simulink model "sampleModel1587"  (R2023a)
settings: Solver=VariableStepAuto  StartTime=0.0  StopTime=10.0  RelTol=1e-3
libraries: hdlsllib x2, simulink x2
settings Model: Creator=user1  LastModifiedBy=user1

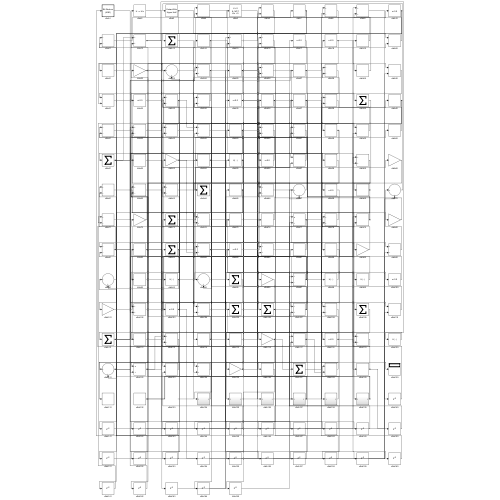
[thumbnail: Simulink's stored preview of the top-level diagram]
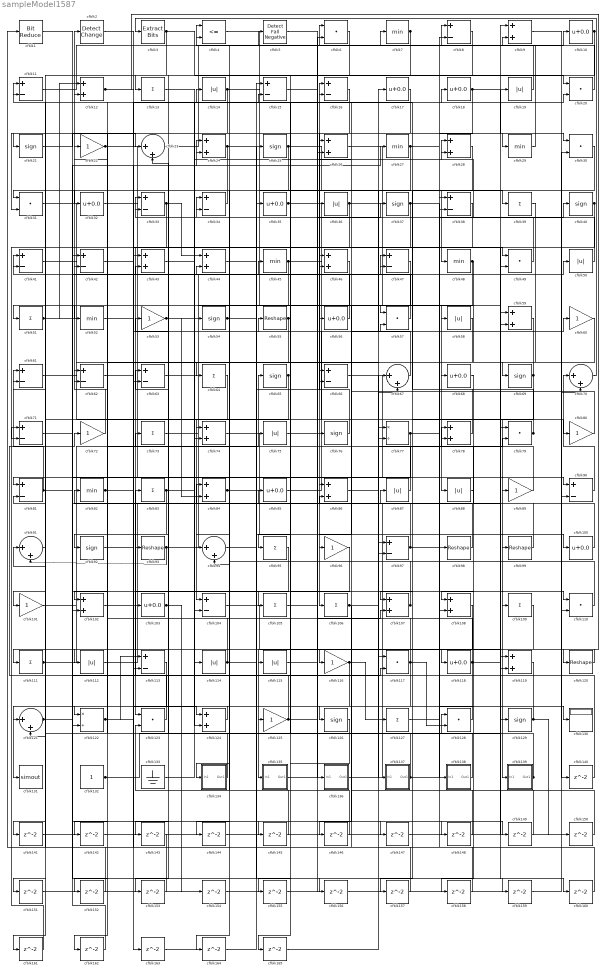
== system sampleModel1587 ==
  cfblk1 : hdlsllib/Logic and Bit Operations/Bit Reduce  mode=AND
  cfblk{10,17..18,32,35,56,68,85,100,103,118} (11 alike) : Bias  Bias=0.0  SaturateOnIntegerOverflow=off
  cfblk{22,53,60,72,80,89,96,101,116,125} (10 alike) : Gain
  cfblk{9,12,24,26,28,43..44,46,59,74,78,84,86,102,107..108,119,124} (18 alike) : Sum
  cfblk{8,11,15..16,33..34,38,41..42,47,61..63,66,71,81,90,97,104,113} (20 alike) : Sum  Inputs=+-
  cfblk{13,39,51,64,73,83,95,105..106,109,111,127} (12 alike) : Sum  Inputs=+
  cfblk{6,20,30..31,49,57,79,110,117,123,128} (11 alike) : DotProduct  OutDataTypeStr=Inherit: Inherit via internal rule
  cfblk{14,19,36,50,58,75,87..88,112,114..115} (11 alike) : Abs  SaturateOnIntegerOverflow=off
  cfblk{55,93,98..99,120} (5 alike) : Reshape
  cfblk{23,67,70,91,94,121} (6 alike) : Sum  Inputs=|++
  cfblk122 : Product  Inputs=*/  RndMeth=Zero  SaturateOnIntegerOverflow=on
  cfblk{21,25,37,40,54,65,69,76,92,126,129} (11 alike) : Signum
  cfblk130 : Display
  cfblk131 : ToWorkspace  VariableName=simout  SaveFormat=Timeseries  SampleTime=-1
  cfblk132 : Constant  SampleTime=-1
  cfblk133 : Ground
  cfblk134 : Subsystem
      settings: LibrarySourceBlock=|
      | hdlsllib/Ports &
      | Subsystems/Subsystem
  cfblk135 : Subsystem
      settings: LibrarySourceBlock=|
      | hdlsllib/Ports &
      | Subsystems/Subsystem
  cfblk136 : Subsystem
      settings: LibrarySourceBlock=|
      | hdlsllib/Ports &
      | Subsystems/Subsystem
  cfblk137 : Subsystem
      settings: LibrarySourceBlock=|
      | hdlsllib/Ports &
      | Subsystems/Subsystem
  cfblk138 : Subsystem
      settings: LibrarySourceBlock=|
      | hdlsllib/Ports &
      | Subsystems/Subsystem
  cfblk139 : Subsystem
      settings: LibrarySourceBlock=|
      | hdlsllib/Ports &
      | Subsystems/Subsystem
  cfblk{140..165} (26 alike) : Delay  SampleTime=1
  cfblk2 : simulink/Logic and Bit Operations/Detect Change  vinit=0  OutDataTypeStr=boolean
      settings: LibrarySourceBlock=|
      | hdlsllib/Logic and Bit
      | Operations/Detect
      | Change
  cfblk{7,27,29,45,48,52,82} (7 alike) : MinMax
  cfblk3 : simulink/Logic and Bit Operations/Extract Bits  bitsToExtract=Upper half  numBits=8  bitIdxRange=[0 7]  outScalingMode=Preserve fixed-point scaling
      settings: LibrarySourceBlock=|
      | hdlsllib/Logic and Bit
      | Operations/Extract Bits
  cfblk4 : RelationalOperator  Operator=<=  OutDataTypeStr=boolean  InputSameDT=off
  cfblk5 : hdlsllib/Logic and Bit Operations/Detect Fall Negative  vinit=0  OutDataTypeStr=boolean
  cfblk77 : Product  Inputs=*/  RndMeth=Zero  SaturateOnIntegerOverflow=on
  wires:
  cfblk33/1 -> cfblk44/1, cfblk52/1
  cfblk14/1 -> cfblk57/1, cfblk31/2
  cfblk87/1 -> cfblk34/1
  cfblk30/1 -> cfblk111/1
  cfblk77/1 -> cfblk81/1, cfblk80/1
  cfblk16/1 -> cfblk106/1
  cfblk139/1(Out1) -> cfblk128/1, cfblk85/1
  cfblk4/1 -> cfblk39/1
  cfblk32/1 -> cfblk90/1
  cfblk26/1 -> cfblk88/1
  cfblk119/1 -> cfblk72/1
  cfblk25/1 -> cfblk134/1(In1), cfblk137/1(In1), cfblk20/2
  cfblk38/1 -> cfblk123/1
  cfblk85/1 -> cfblk60/1
  cfblk76/1 -> cfblk16/1
  cfblk128/1 -> cfblk126/1
  cfblk36/1 -> cfblk58/1, cfblk71/2
  cfblk28/1 -> cfblk48/1
  cfblk111/1 -> cfblk87/1, cfblk27/1, cfblk84/1
  cfblk115/1 -> cfblk76/1
  cfblk27/1 -> cfblk31/1, cfblk29/1
  cfblk43/1 -> cfblk18/1
  cfblk35/1 -> cfblk139/1(In1), cfblk97/2
  cfblk73/1 -> cfblk38/2
  cfblk57/1 -> cfblk11/1
  cfblk129/1 -> cfblk83/1, cfblk150/1
  cfblk125/1 -> cfblk81/2, cfblk107/2
  cfblk70/1 -> cfblk3/1
  cfblk72/1 -> cfblk2/1
  cfblk37/1 -> cfblk130/1, cfblk93/1, cfblk107/1
  cfblk101/1 -> cfblk65/1
  cfblk105/1 -> cfblk47/1
  cfblk65/1 -> cfblk104/1, cfblk94/2
  cfblk117/1 -> cfblk12/2, cfblk128/2, cfblk144/1
  cfblk10/1 -> cfblk95/1, cfblk113/2
  cfblk98/1 -> cfblk45/1
  cfblk104/1 -> cfblk116/1
  cfblk56/1 -> cfblk36/1
  cfblk116/1 -> cfblk127/1, cfblk153/1
  cfblk100/1 -> cfblk78/1
  cfblk8/1 -> cfblk13/1
  cfblk66/1 -> cfblk138/1(In1)
  cfblk13/1 -> cfblk114/1
  cfblk12/1 -> cfblk120/1, cfblk105/1
  cfblk81/1 -> cfblk61/1, cfblk89/1, cfblk145/1
  cfblk91/1 -> cfblk41/1
  cfblk46/1 -> cfblk51/1
  cfblk31/1 -> cfblk104/2
  cfblk53/1 -> cfblk56/1, cfblk84/2
  cfblk113/1 -> cfblk131/1
  cfblk136/1(Out1) -> cfblk9/1
  cfblk132/1 -> cfblk59/1, cfblk6/2
  cfblk89/1 -> cfblk22/1
  cfblk124/1 -> cfblk121/1
  cfblk22/1 -> cfblk119/1, cfblk14/1
  cfblk110/1 -> cfblk15/2
  cfblk7/1 -> cfblk121/2, cfblk143/1
  cfblk108/1 -> cfblk135/1(In1)
  cfblk5/1 -> cfblk136/1(In1)
  cfblk103/1 -> cfblk63/1, cfblk154/1
  cfblk59/1 -> cfblk122/1
  cfblk107/1 -> cfblk82/1, cfblk75/1
  cfblk133/1 -> cfblk28/1
  cfblk67/1 -> cfblk26/1
  cfblk102/1 -> cfblk19/1
  cfblk45/1 -> cfblk59/2, cfblk102/2, cfblk152/1
  cfblk112/1 -> cfblk77/2
  cfblk82/1 -> cfblk124/1, cfblk24/1
  cfblk93/1 -> cfblk57/2, cfblk91/2
  cfblk78/1 -> cfblk47/2
  cfblk60/1 -> cfblk124/2
  cfblk127/1 -> cfblk10/1
  cfblk41/1 -> cfblk43/2
  cfblk2/1 -> cfblk74/1
  cfblk55/1 -> cfblk115/1, cfblk64/1
  cfblk15/1 -> cfblk8/1
  cfblk83/1 -> cfblk54/1, cfblk92/1
  cfblk44/1 -> cfblk86/1
  cfblk135/1(Out1) -> cfblk37/1
  cfblk23/1 -> cfblk7/1
  cfblk50/1 -> cfblk28/2
  cfblk134/1(Out1) -> cfblk62/1
  cfblk58/1 -> cfblk102/1
  cfblk138/1(Out1) -> cfblk53/1
  cfblk63/1 -> cfblk17/1
  cfblk75/1 -> cfblk118/1
  cfblk18/1 -> cfblk63/2, cfblk30/1
  cfblk90/1 -> cfblk70/1
  cfblk3/1 -> cfblk21/1, cfblk20/1
  cfblk42/1 -> cfblk49/1
  cfblk24/1 -> cfblk74/2, cfblk159/1
  cfblk121/1 -> cfblk117/2, cfblk156/1
  cfblk29/1 -> cfblk9/2
  cfblk95/1 -> cfblk103/1
  cfblk96/1 -> cfblk125/1
  cfblk6/1 -> cfblk101/1
  cfblk99/1 -> cfblk78/2
  cfblk52/1 -> cfblk109/1
  cfblk49/1 -> cfblk33/1
  cfblk54/1 -> cfblk94/1, cfblk147/1
  cfblk61/1 -> cfblk98/1
  cfblk97/1 -> cfblk40/1, cfblk33/2, cfblk4/2, cfblk62/2
  cfblk123/1 -> cfblk42/2
  cfblk79/1 -> cfblk11/2, cfblk46/1
  cfblk88/1 -> cfblk108/1
  cfblk86/1 -> cfblk79/2
  cfblk137/1(Out1) -> cfblk108/2, cfblk34/2, cfblk61/2
  cfblk34/1 -> cfblk32/1
  cfblk114/1 -> cfblk73/1, cfblk66/2
  cfblk74/1 -> cfblk129/1
  cfblk48/1 -> cfblk68/1, cfblk96/1
  cfblk80/1 -> cfblk16/2
  cfblk1/1 -> cfblk110/1
  cfblk20/1 -> cfblk4/1
  cfblk40/1 -> cfblk164/1, cfblk165/1
  cfblk39/1 -> cfblk69/1
  cfblk106/1 -> cfblk119/2, cfblk146/1
  cfblk84/1 -> cfblk99/1, cfblk100/1
  cfblk19/1 -> cfblk6/1
  cfblk11/1 -> cfblk5/1
  cfblk120/1 -> cfblk112/1
  cfblk71/1 -> cfblk50/1
  cfblk69/1 -> cfblk66/1, cfblk157/1
  cfblk51/1 -> cfblk67/2, cfblk12/1, cfblk24/2, cfblk141/1
  cfblk122/1 -> cfblk55/1, cfblk113/1
  cfblk118/1 -> cfblk23/2, cfblk160/1, cfblk161/1
  cfblk47/1 -> cfblk122/2
  cfblk21/1 -> cfblk23/1
  cfblk9/1 -> cfblk140/1
  cfblk140/1 -> cfblk79/1
  cfblk141/1 -> cfblk49/2
  cfblk17/1 -> cfblk142/1
  cfblk142/1 -> cfblk15/1
  cfblk143/1 -> cfblk1/1
  cfblk144/1 -> cfblk90/2
  cfblk145/1 -> cfblk44/2
  cfblk146/1 -> cfblk123/2
  cfblk147/1 -> cfblk8/2
  cfblk94/1 -> cfblk148/1
  cfblk148/1 -> cfblk117/1
  cfblk92/1 -> cfblk149/1
  cfblk149/1 -> cfblk77/1
  cfblk150/1 -> cfblk46/2
  cfblk64/1 -> cfblk151/1
  cfblk151/1 -> cfblk110/2
  cfblk152/1 -> cfblk91/1
  cfblk153/1 -> cfblk43/1
  cfblk154/1 -> cfblk26/2
  cfblk126/1 -> cfblk155/1
  cfblk155/1 -> cfblk67/1
  cfblk156/1 -> cfblk70/2
  cfblk157/1 -> cfblk41/2
  cfblk68/1 -> cfblk158/1
  cfblk158/1 -> cfblk38/1
  cfblk159/1 -> cfblk30/2
  cfblk160/1 -> cfblk86/2
  cfblk161/1 -> cfblk71/1
  cfblk109/1 -> cfblk162/1
  cfblk162/1 -> cfblk42/1
  cfblk62/1 -> cfblk163/1
  cfblk163/1 -> cfblk25/1
  cfblk164/1 -> cfblk35/1
  cfblk165/1 -> cfblk97/1

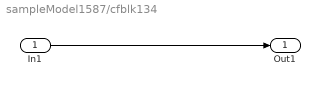
== system sampleModel1587/cfblk134 ==
  In1 : Inport
  Out1 : Outport
  wires:
  In1/1 -> Out1/1

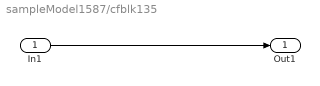
== system sampleModel1587/cfblk135 ==
  In1 : Inport
  Out1 : Outport
  wires:
  In1/1 -> Out1/1

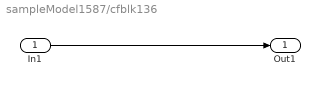
== system sampleModel1587/cfblk136 ==
  In1 : Inport
  Out1 : Outport
  wires:
  In1/1 -> Out1/1

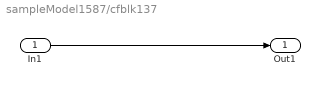
== system sampleModel1587/cfblk137 ==
  In1 : Inport
  Out1 : Outport
  wires:
  In1/1 -> Out1/1

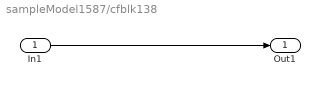
== system sampleModel1587/cfblk138 ==
  In1 : Inport
  Out1 : Outport
  wires:
  In1/1 -> Out1/1

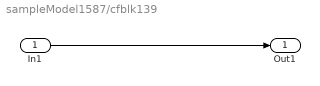
== system sampleModel1587/cfblk139 ==
  In1 : Inport
  Out1 : Outport
  wires:
  In1/1 -> Out1/1
